simulink model "swing_flexion_test"  (R2019b)
settings: Solver=VariableStepAuto  StartTime=0.0  StopTime=3  FixedStep=0.0002  MaxStep=0.01
PostLoadFcn:
  | vertGRF_entry_avg   =9;
  | horGRF_entry_avg    = vertGRF_entry_avg + 2;
  | % Import the data from Excel for a lookup table
  | data = xlsread('../Plot_figures/winterdata.xlsx','Ft snf');
  | % Row indices for lookup table
  | breakpoints1 = data(1:51,1);
  | % Column indices for lookup table
  | %breakpoints2 = data(1,2:end);
  | % Output values for lookup table
  | vertGRF_avg         = data(1:max(size(breakpoints1)),vertGRF_entry_avg);
  | horGRF_avg          = data(1:max(size(breakpoints1)),horGRF_entry_avg);
InitFcn:
  | Prosthesis3R60Params;
values from neighbouring files (symbols this model uses):
  dt_visual = 0.001    [Prosthesis3R60Params.m]
  j12_i_0 = 73.55    [Prosthesis3R60Params.m]
  j15_i_0 = 90    [Prosthesis3R60Params.m]
  j9_i_0 = -99.5    [Prosthesis3R60Params.m]
  J_shank = m_shank*L_shank^2/12    (= 0.001125)    [Prosthesis3R60Params.m]
  J_thigh = m_thigh*L_thigh^2/12    (= 0.06)    [Prosthesis3R60Params.m]
  L_shank = 0.3    [Prosthesis3R60Params.m]
  L_thigh = 0.3    [Prosthesis3R60Params.m]
  m_shank = 150*1e-3    (= 0.15)    [Prosthesis3R60Params.m]
  m_thigh = 8    [Prosthesis3R60Params.m]
undefined symbols (not defined in the file or in its folder): X, Y, Z
libraries: sm_lib x16, nesl_utility x2, NeuroMuscularLibrary x1, smdoc_compound_rigid_bodies x1
settings Model: PacingRate=0.056000  OrderedModelArguments=off  Creator=Nathan  LastModifiedBy=Nathan
settings DataIOCC: ReturnWorkspaceOutputs=off

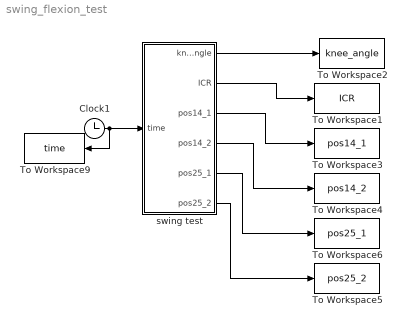
== system swing_flexion_test ==
  Clock1 : Clock
  To Workspace1 : ToWorkspace  VariableName=ICR  SampleTime=dt_visual
  To Workspace2 : ToWorkspace  VariableName=knee_angle  SampleTime=dt_visual
  To Workspace3 : ToWorkspace  VariableName=pos14_1  SampleTime=dt_visual
  To Workspace4 : ToWorkspace  VariableName=pos14_2  SampleTime=dt_visual
  To Workspace5 : ToWorkspace  VariableName=pos25_2  SampleTime=dt_visual
  To Workspace6 : ToWorkspace  VariableName=pos25_1  SampleTime=dt_visual
  To Workspace9 : ToWorkspace  VariableName=time  SampleTime=dt_visual
  swing test : Subsystem  mask{j9_i=j9_i_0, j12_i=j12_i_0, j15_i=j15_i_0}
      mask prompts: j9_i "Initial angle joint 9"; j12_i "Initial angle joint 12"; j15_i "Initial angle joint 15"
  wires:
  swing test/1(knee_angle) -> To Workspace2/1
  swing test/4(pos14_2) -> To Workspace4/1
  swing test/2(ICR) -> To Workspace1/1
  swing test/3(pos14_1) -> To Workspace3/1
  swing test/5(pos25_1) -> To Workspace6/1
  swing test/6(pos25_2) -> To Workspace5/1
  Clock1/1 -> To Workspace9/1, swing test/1(time)

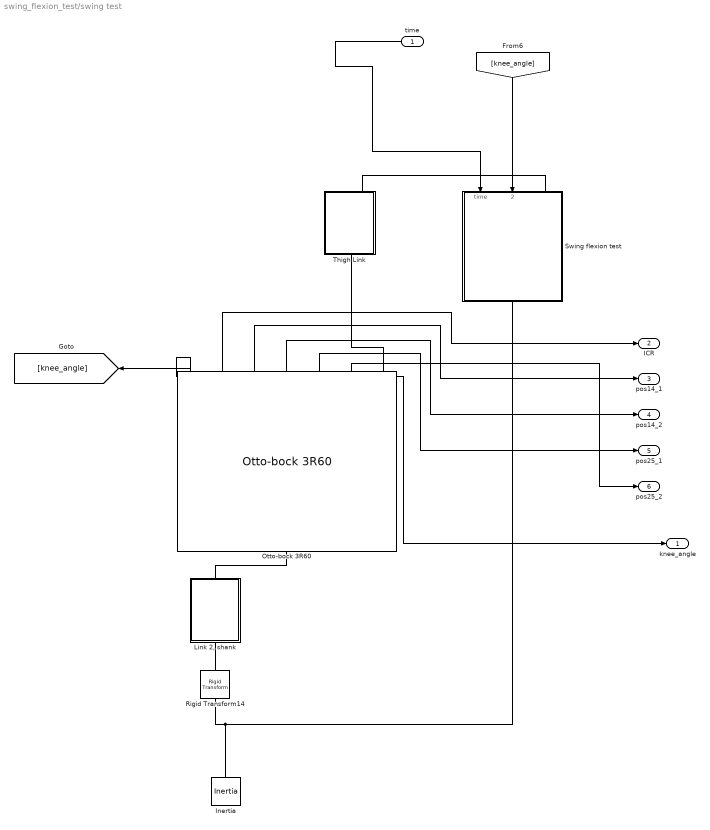
== system swing_flexion_test/swing test ==
  time : Inport
  Inertia : sm_lib/Body Elements/Inertia  InertiaType=PointMass  Mass=1  MassUnits=kg  CenterOfMass=[0 0 0]  CenterOfMassUnits=m  MomentsOfInertia=[1 1 1]  MomentsOfInertiaUnits=kg*m^2  ProductsOfInertia=[0 0 0]  ProductsOfInertiaUnits=kg*m^2  GraphicType=Marker  MarkerShape=Inertia  MarkerSize=5  GraphicVisPropType=SimpleVisualProperties  GraphicDiffuseColor=[0.5 0.5 0.5]  GraphicSpecularColor=[0.5 0.5 0.5 1.0]  GraphicAmbientColor=[0.15 0.15 0.15 1.0]  GraphicEmissiveColor=[0.0 0.0 0.0 1.0]  GraphicShininess=75  GraphicOpacity=1.0
  "Link 2, shank" : Subsystem  mask{L=L_shank, W=0.2/100, T=0.08/100, R=0.005/100, m=m_shank, LinkRGB=[84 130 53]./255, PegRGB=[1 0.6 0.25], J=J_shank}
      mask prompts: L "Length"; W "Width"; T "Thickness"; R "Peg Radius"; m "Mass"; LinkRGB "Link Color"; PegRGB "Peg Color"; J "Moment of Inertia"
      mask init:
      | % Cross-section of main:
      | Alpha = (-pi/2:0.01:pi/2)';
      | Beta = (pi/2:-0.01:-pi/2)';
      | PegCS = [L/2+W/2*cos(Alpha)... 
      | W/2*sin(Alpha)];
      | HoleCS = [-L/2 W/2; -L/2 + R*cos(Beta)... 
      | R*sin(Beta); -L/2 -W/2];
      | MainCS = [PegCS; HoleCS];
      | 
      | % Cross-section of hole:
      | Alpha = (pi/2:0.01:3*pi/2)';
      | Beta = (3*pi/2:-0.01:pi/2)';
      | HoleCS = [W/2*cos(Alpha) W/2*sin(Alpha);
      | R*cos(Beta) R*sin(Beta)];
  Otto-bock 3R60 : NeuroMuscularLibrary/Otto-bock 3R60  SystemSampleTime=-1  Latency=0  AutoFrameSizeCalculation=off
  Rigid Transform14 : sm_lib/Frames and Transforms/Rigid Transform  TranslationMethod=None  TranslationStandardOffset=0  TranslationLengthUnit=m  TranslationStandardAxis=+Z  TranslationCartesianOffset=[0 0 0]  TranslationROffset=0  TranslationROffsetUnits=m  TranslationZOffset=0  TranslationZOffsetUnits=m  TranslationThetaOffset=0  TranslationThetaOffsetUnits=deg  RotationMethod=StandardAxis  RotationAngleUnits=deg  RotationStandardAxis=+Z  RotationAngle=180  RotationArbitraryAxis=[0 0 1]  FollAlignAxisA=+X  BaseAlignAxisA=+Y  FollAlignAxisB=+Y  BaseAlignAxisB=+Z  RotationSequenceAxes=FollowerAxes  RotationSequence=XYX  RotationSequenceAngles=[0 0 0]  RotationSequenceAnglesUnits=deg  RotationMatrix=[1 0 0; 0 1 0; 0 0 1]
  Swing flexion test : Subsystem
  Thigh Link : Subsystem  mask{L=L_thigh, W=0.2/100, T=0.08/100, R=0.005/100, m=m_thigh, LinkRGB=[68 114 196]./255, PegRGB=[1 0.6 0.25], J=J_thigh}
      mask prompts: L "Length"; W "Width"; T "Thickness"; R "Peg Radius"; m "Mass"; LinkRGB "Link Color"; PegRGB "Peg Color"; J "Moment of Inertia"
      mask init: same as swing_flexion_test/swing test/Link 2, shank
  knee_angle : Outport
  ICR : Outport  Port=2
  pos14_1 : Outport  Port=3
  pos14_2 : Outport  Port=4
  pos25_1 : Outport  Port=5
  pos25_2 : Outport  Port=6
  wires:
  Otto-bock 3R60/1 -> [knee_angle], knee_angle/1
  Otto-bock 3R60/2 -> ICR/1
  [knee_angle] -> Swing flexion test/2(Knee angle)
  Otto-bock 3R60/3 -> pos14_1/1
  time/1 -> Swing flexion test/1(time)
  Otto-bock 3R60/4 -> pos14_2/1
  Otto-bock 3R60/5 -> pos25_1/1
  Otto-bock 3R60/6 -> pos25_2/1
  connections:
  Otto-bock 3R60/RConn1 -- Thigh Link/LConn1
  Rigid Transform14/LConn1 -- Swing flexion test/RConn1 -- Inertia/RConn1
  Swing flexion test/LConn1 -- Thigh Link/RConn2
  Rigid Transform14/RConn1 -- "Link 2, shank"/LConn1
  "Link 2, shank"/RConn1 -- Otto-bock 3R60/LConn1

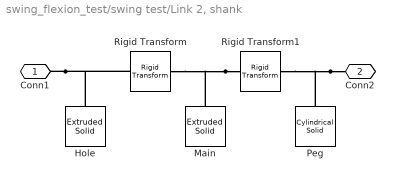
== system swing_flexion_test/swing test/Link 2, shank ==
  Hole : sm_lib/Body Elements/Extruded Solid  GraphicAmbientColor=[0.15 0.15 0.15 1.0]  BasedOnType=Density  CenterOfMass=[0 0 0]  CenterOfMassUnits=m  GraphicDiffuseColor=LinkRGB  ExtrusionCrossSection=HoleCS  ExtrusionCrossSectionUnits=m  Density=0  DensityUnits=kg/(m^3)  DoExposeReferenceFrame=on  GraphicEmissiveColor=[0.0 0.0 0.0 1.0]  ExportEntireGeometry=off  ExtrusionLength=T  ExtrusionLengthUnits=m  ExtrusionType=General  SerializedFrames=<Frames/>  MarkerShape=Sphere  MarkerSize=10  GraphicType=FromGeometry  InertiaType=PointMass  Mass=0  MassUnits=kg  MomentsOfInertia=[1 1 1]  MomentsOfInertiaUnits=kg*m^2  PolygonNumSides=3  GraphicOpacity=1.0  PolygonOuterRadius=1  PolygonOuterRadiusUnits=m  ProductsOfInertia=[0 0 0]  ProductsOfInertiaUnits=kg*m^2  GraphicShininess=75  GraphicSpecularColor=[0.5 0.5 0.5 1.0]  GraphicVisPropType=SimpleVisualProperties
      settings: SourceProductName=Simscape Multibody
  Main : sm_lib/Body Elements/Extruded Solid  GraphicAmbientColor=[0.15 0.15 0.15 1.0]  BasedOnType=Density  CenterOfMass=[0 0 0]  CenterOfMassUnits=m  GraphicDiffuseColor=LinkRGB  ExtrusionCrossSection=MainCS  ExtrusionCrossSectionUnits=m  Density=0  DensityUnits=kg/(m^3)  DoExposeReferenceFrame=on  GraphicEmissiveColor=[0.0 0.0 0.0 1.0]  ExportEntireGeometry=off  ExtrusionLength=T  ExtrusionLengthUnits=m  ExtrusionType=General  SerializedFrames=<Frames/>  MarkerShape=Sphere  MarkerSize=10  GraphicType=FromGeometry  InertiaType=Custom  Mass=m  MassUnits=kg  MomentsOfInertia=[0 0 J]  MomentsOfInertiaUnits=kg*m^2  PolygonNumSides=3  GraphicOpacity=1.0  PolygonOuterRadius=1  PolygonOuterRadiusUnits=m  ProductsOfInertia=[0 0 0]  ProductsOfInertiaUnits=kg*m^2  GraphicShininess=75  GraphicSpecularColor=[0.5 0.5 0.5 1.0]  GraphicVisPropType=SimpleVisualProperties
      settings: SourceProductName=Simscape Multibody
  Peg : sm_lib/Body Elements/Cylindrical Solid  GraphicAmbientColor=[0.15 0.15 0.15 1.0]  BasedOnType=Mass  CenterOfMass=[0 0 0]  CenterOfMassUnits=m  GraphicDiffuseColor=PegRGB  CylinderLength=2*T  CylinderLengthUnits=m  CylinderRadius=R  CylinderRadiusUnits=m  Density=0  DensityUnits=kg/(m^3)  DoExposeReferenceFrame=on  GraphicEmissiveColor=[0.0 0.0 0.0 1.0]  ExportEntireGeometry=off  SerializedFrames=<Frames/>  MarkerShape=Sphere  MarkerSize=10  GraphicType=FromGeometry  InertiaType=PointMass  Mass=0  MassUnits=kg  MomentsOfInertia=[1 1 1]  MomentsOfInertiaUnits=kg*m^2  GraphicOpacity=1.0  ProductsOfInertia=[0 0 0]  ProductsOfInertiaUnits=kg*m^2  GraphicShininess=75  GraphicSpecularColor=[0.5 0.5 0.5 1.0]  GraphicVisPropType=SimpleVisualProperties
  Rigid Transform : sm_lib/Frames and Transforms/Rigid Transform  TranslationMethod=StandardAxis  TranslationStandardOffset=L/2  TranslationLengthUnit=m  TranslationStandardAxis=-X  TranslationCartesianOffset=[0 0 0]  TranslationROffset=0  TranslationROffsetUnits=m  TranslationZOffset=0  TranslationZOffsetUnits=m  TranslationThetaOffset=0  TranslationThetaOffsetUnits=deg  RotationMethod=None  RotationAngleUnits=deg  RotationStandardAxis=+Z  RotationAngle=0  RotationArbitraryAxis=[0 0 1]  FollAlignAxisA=+X  BaseAlignAxisA=+Y  FollAlignAxisB=+Y  BaseAlignAxisB=+Z  RotationSequenceAxes=FollowerAxes  RotationSequence=XYX  RotationSequenceAngles=[0 0 0]  RotationSequenceAnglesUnits=deg  RotationMatrix=[1 0 0; 0 1 0; 0 0 1]
  Rigid Transform1 : sm_lib/Frames and Transforms/Rigid Transform  TranslationMethod=Cartesian  TranslationStandardOffset=0  TranslationLengthUnit=m  TranslationStandardAxis=+X  TranslationCartesianOffset=[L/2 0 3/2*T]  TranslationROffset=0  TranslationROffsetUnits=m  TranslationZOffset=0  TranslationZOffsetUnits=m  TranslationThetaOffset=0  TranslationThetaOffsetUnits=deg  RotationMethod=None  RotationAngleUnits=deg  RotationStandardAxis=+Z  RotationAngle=0  RotationArbitraryAxis=[0 0 1]  FollAlignAxisA=+X  BaseAlignAxisA=+Y  FollAlignAxisB=+Y  BaseAlignAxisB=+Z  RotationSequenceAxes=FollowerAxes  RotationSequence=XYX  RotationSequenceAngles=[0 0 0]  RotationSequenceAnglesUnits=deg  RotationMatrix=[1 0 0; 0 1 0; 0 0 1]
  Conn1 : PMIOPort  Side=Left
  Conn2 : PMIOPort  Port=2  Side=Right
  connections:
  Rigid Transform1/LConn1 -- Main/RConn1 -- Rigid Transform/LConn1
  Conn1/RConn1 -- Rigid Transform/RConn1 -- Hole/RConn1
  Conn2/RConn1 -- Rigid Transform1/RConn1 -- Peg/RConn1

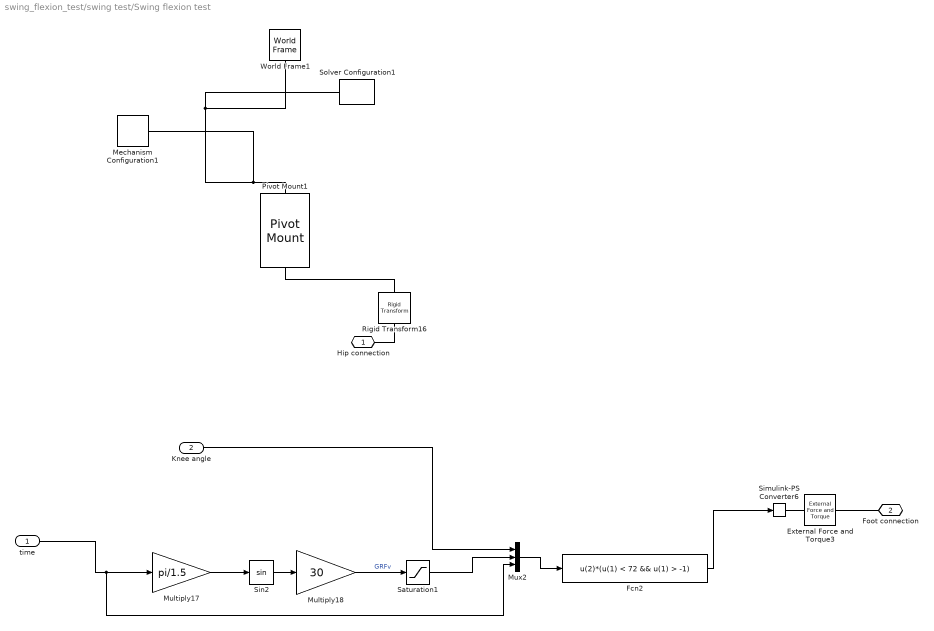
== system swing_flexion_test/swing test/Swing flexion test ==
  time : Inport
  Knee angle : Inport  Port=2
  External Force and Torque3 : sm_lib/Forces and Torques/External Force and Torque  ForceResolutionFrame=AttachedFrame  EnableForceX=off  EnableForceY=on  EnableForceZ=off  EnableForce=off  TorqueResolutionFrame=AttachedFrame  EnableTorqueX=off  EnableTorqueY=off  EnableTorqueZ=off  EnableTorque=off
  Fcn2 : Fcn  Expr=u(2)*(u(1) < 72 && u(1) > -1)
  Mechanism Configuration1 : sm_lib/Utilities/Mechanism Configuration  UniformGravity=Constant  GravityVector=[0 0 -9.80665]  GravityUnits=m/s^2  LinearizationDelta=0.001
  Multiply17 : Gain  Gain=pi/1.5
  Multiply18 : Gain  Gain=30
  Mux2 : Mux  Inputs=3
  Pivot Mount1 : smdoc_compound_rigid_bodies/Pivot Mount  HexagonR=0.4/100  T=0.08/100  Rho=0  HexagonRGB=[0.25 0.4 0.7]  PegR=0.005/100  PegRGB=[1 0.6 0.25]
      link override Hexagon: ExtrusionLengthUnits=m  PolygonOuterRadiusUnits=m
      link override Peg: CylinderLengthUnits=m  CylinderRadiusUnits=m
      link override To Peg: TranslationLengthUnit=m
  Rigid Transform16 : sm_lib/Frames and Transforms/Rigid Transform  TranslationMethod=None  TranslationStandardOffset=0  TranslationLengthUnit=m  TranslationStandardAxis=+Z  TranslationCartesianOffset=[0 0 0]  TranslationROffset=0  TranslationROffsetUnits=m  TranslationZOffset=0  TranslationZOffsetUnits=m  TranslationThetaOffset=0  TranslationThetaOffsetUnits=deg  RotationMethod=StandardAxis  RotationAngleUnits=deg  RotationStandardAxis=+Z  RotationAngle=180  RotationArbitraryAxis=[0 0 1]  FollAlignAxisA=+X  BaseAlignAxisA=+Y  FollAlignAxisB=+Y  BaseAlignAxisB=+Z  RotationSequenceAxes=FollowerAxes  RotationSequence=XYX  RotationSequenceAngles=[0 0 0]  RotationSequenceAnglesUnits=deg  RotationMatrix=[1 0 0; 0 1 0; 0 0 1]
  Saturation1 : Saturate  UpperLimit=inf  LowerLimit=0  ZeroCross=off
  Simulink-PS Converter6 : nesl_utility/Simulink-PS Converter  PhysicalDomain=network_engine_domain  SubClassName=ps_input  LeftPortType=input  RightPortType=output  PseudoPeriodic=off  Frequencies=[]  NoiseDistribution=none  NoiseParameters=[]  Unit=N  AffineConversion=off  FilteringAndDerivatives=provide  SimscapeFilterOrder=1  InputFilterTimeConstant=0.001  UdotUserProvided=0
  Sin2 : Trigonometry
  Solver Configuration1 : nesl_utility/Solver Configuration  PhysicalDomain=network_engine_domain  SubClassName=solver  LeftPortType=input  RightPortType=generic  Tones=[]  Harmonics=[]  SimulateNoise=off  Profile=off  UseLocalSampling=off  EnableSwitchedLinearOptims=on  FrequencyDomain=off  UseCCode=off  RelTol=0.001  AbsTol=1e-06  MinStep=1e-09  ToWorkspace=off  RevertToSquareIcSolve=off  NumHomotopyIterations=100  PhasorMode=off  PhasorModeNumHarmonics=1  DoDC=off  ResidualTolerance=1e-09  UseLocalSolver=off  LocalSolverChoice=NE_BACKWARD_EULER_ADVANCER  LocalSolverSampleTime=0.001  DoFixedCost=off  MaxNonlinIter=3  MaxModeIter=2  LinearAlgebra=Sparse  EquationFormulation=NE_TIME_EF  DelaysMemoryBudget=1024  AutomaticFiltering=on  FilteringTimeConstant=0.001  PartitionStorageMethod=AS_NEEDED  PartitionMemoryBudget=1024  PartitionMethod=ROBUST
  World Frame1 : sm_lib/Frames and Transforms/World Frame
  Hip connection : PMIOPort  Side=Left
  Foot connection : PMIOPort  Port=2  Side=Right
  wires:
  Knee angle/1 -> Mux2/1
  Sin2/1 -> Multiply18/1
  Saturation1/1 -> Mux2/2
  Multiply18/1 -> Saturation1/1  "GRFv"
  Multiply17/1 -> Sin2/1
  Fcn2/1 -> Simulink-PS Converter6/1
  Mux2/1 -> Fcn2/1
  time/1 -> Mux2/3, Multiply17/1
  connections:
  Simulink-PS Converter6/RConn1 -- External Force and Torque3/LConn1
  Rigid Transform16/RConn1 -- Pivot Mount1/RConn1
  Solver Configuration1/RConn1 -- Pivot Mount1/LConn1 -- Mechanism Configuration1/RConn1 -- World Frame1/RConn1
  Rigid Transform16/LConn1 -- Hip connection/RConn1
  External Force and Torque3/RConn1 -- Foot connection/RConn1

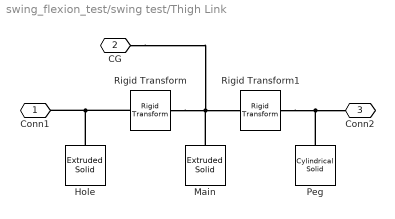
== system swing_flexion_test/swing test/Thigh Link ==
  Hole : sm_lib/Body Elements/Extruded Solid  GraphicAmbientColor=[0.15 0.15 0.15 1.0]  BasedOnType=Density  CenterOfMass=[0 0 0]  CenterOfMassUnits=m  GraphicDiffuseColor=LinkRGB  ExtrusionCrossSection=HoleCS  ExtrusionCrossSectionUnits=m  Density=0  DensityUnits=kg/(m^3)  DoExposeReferenceFrame=on  GraphicEmissiveColor=[0.0 0.0 0.0 1.0]  ExportEntireGeometry=off  ExtrusionLength=T  ExtrusionLengthUnits=m  ExtrusionType=General  SerializedFrames=<Frames/>  MarkerShape=Sphere  MarkerSize=10  GraphicType=FromGeometry  InertiaType=PointMass  Mass=0  MassUnits=kg  MomentsOfInertia=[1 1 1]  MomentsOfInertiaUnits=kg*m^2  PolygonNumSides=3  GraphicOpacity=1.0  PolygonOuterRadius=1  PolygonOuterRadiusUnits=m  ProductsOfInertia=[0 0 0]  ProductsOfInertiaUnits=kg*m^2  GraphicShininess=75  GraphicSpecularColor=[0.5 0.5 0.5 1.0]  GraphicVisPropType=SimpleVisualProperties
      settings: SourceProductName=Simscape Multibody
  Main : sm_lib/Body Elements/Extruded Solid  GraphicAmbientColor=[0.15 0.15 0.15 1.0]  BasedOnType=Density  CenterOfMass=[0 0 0]  CenterOfMassUnits=m  GraphicDiffuseColor=LinkRGB  ExtrusionCrossSection=MainCS  ExtrusionCrossSectionUnits=m  Density=0  DensityUnits=kg/(m^3)  DoExposeReferenceFrame=on  GraphicEmissiveColor=[0.0 0.0 0.0 1.0]  ExportEntireGeometry=off  ExtrusionLength=T  ExtrusionLengthUnits=m  ExtrusionType=General  SerializedFrames=<Frames/>  MarkerShape=Sphere  MarkerSize=10  GraphicType=FromGeometry  InertiaType=Custom  Mass=m  MassUnits=kg  MomentsOfInertia=[0 0 J]  MomentsOfInertiaUnits=kg*m^2  PolygonNumSides=3  GraphicOpacity=1.0  PolygonOuterRadius=1  PolygonOuterRadiusUnits=m  ProductsOfInertia=[0 0 0]  ProductsOfInertiaUnits=kg*m^2  GraphicShininess=75  GraphicSpecularColor=[0.5 0.5 0.5 1.0]  GraphicVisPropType=SimpleVisualProperties
      settings: SourceProductName=Simscape Multibody
  Peg : sm_lib/Body Elements/Cylindrical Solid  GraphicAmbientColor=[0.15 0.15 0.15 1.0]  BasedOnType=Density  CenterOfMass=[0 0 0]  CenterOfMassUnits=m  GraphicDiffuseColor=PegRGB  CylinderLength=2*T  CylinderLengthUnits=m  CylinderRadius=R  CylinderRadiusUnits=m  Density=0  DensityUnits=kg/(m^3)  DoExposeReferenceFrame=on  GraphicEmissiveColor=[0.0 0.0 0.0 1.0]  ExportEntireGeometry=off  SerializedFrames=<Frames/>  MarkerShape=Sphere  MarkerSize=10  GraphicType=FromGeometry  InertiaType=PointMass  Mass=0  MassUnits=kg  MomentsOfInertia=[1 1 1]  MomentsOfInertiaUnits=kg*m^2  GraphicOpacity=1.0  ProductsOfInertia=[0 0 0]  ProductsOfInertiaUnits=kg*m^2  GraphicShininess=75  GraphicSpecularColor=[0.5 0.5 0.5 1.0]  GraphicVisPropType=SimpleVisualProperties
  Rigid Transform : sm_lib/Frames and Transforms/Rigid Transform  TranslationMethod=StandardAxis  TranslationStandardOffset=L/2  TranslationLengthUnit=m  TranslationStandardAxis=-X  TranslationCartesianOffset=[0 0 0]  TranslationROffset=0  TranslationROffsetUnits=m  TranslationZOffset=0  TranslationZOffsetUnits=m  TranslationThetaOffset=0  TranslationThetaOffsetUnits=deg  RotationMethod=None  RotationAngleUnits=deg  RotationStandardAxis=+Z  RotationAngle=0  RotationArbitraryAxis=[0 0 1]  FollAlignAxisA=+X  BaseAlignAxisA=+Y  FollAlignAxisB=+Y  BaseAlignAxisB=+Z  RotationSequenceAxes=FollowerAxes  RotationSequence=XYX  RotationSequenceAngles=[0 0 0]  RotationSequenceAnglesUnits=deg  RotationMatrix=[1 0 0; 0 1 0; 0 0 1]
  Rigid Transform1 : sm_lib/Frames and Transforms/Rigid Transform  TranslationMethod=Cartesian  TranslationStandardOffset=0  TranslationLengthUnit=m  TranslationStandardAxis=+X  TranslationCartesianOffset=[L/2 0 3/2*T]  TranslationROffset=0  TranslationROffsetUnits=m  TranslationZOffset=0  TranslationZOffsetUnits=m  TranslationThetaOffset=0  TranslationThetaOffsetUnits=deg  RotationMethod=None  RotationAngleUnits=deg  RotationStandardAxis=+Z  RotationAngle=0  RotationArbitraryAxis=[0 0 1]  FollAlignAxisA=+X  BaseAlignAxisA=+Y  FollAlignAxisB=+Y  BaseAlignAxisB=+Z  RotationSequenceAxes=FollowerAxes  RotationSequence=XYX  RotationSequenceAngles=[0 0 0]  RotationSequenceAnglesUnits=deg  RotationMatrix=[1 0 0; 0 1 0; 0 0 1]
  Conn1 : PMIOPort  Side=Left
  CG : PMIOPort  Port=2  Side=Right
  Conn2 : PMIOPort  Port=3  Side=Right
  connections:
  Peg/RConn1 -- Rigid Transform1/RConn1 -- Conn2/RConn1
  Hole/RConn1 -- Rigid Transform/RConn1 -- Conn1/RConn1
  Rigid Transform/LConn1 -- CG/RConn1 -- Main/RConn1 -- Rigid Transform1/LConn1
